simulink library "mobileRoboticsTrainingLib"  (R2017a)
settings: Solver=FixedStepDiscrete  StartTime=0.0  StopTime=10.0  FixedStep=0.01  RelTol=1e-3
values from neighbouring files (symbols this model uses):
  lineLength = xAxesLim(2)/15    [setupRobotSim.m]
  mapForSim = evalin('base',mapVar)    [setStartingPoint.m]    (also in setupRobotSim.m)
undefined symbols (not defined in the file or in its folder): DiscIntNeverNeededParam
libraries: cstblocks x1, simulink_extras x1, simulink x1
settings Model: Creator=sseshadr  LastModifiedBy=sseshadr

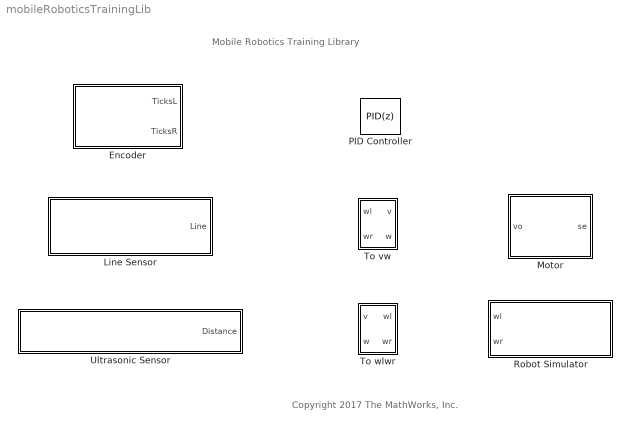
== system mobileRoboticsTrainingLib ==
  note: Mobile Robotics Training Library
  note: Copyright 2017 The MathWorks, Inc.
  Encoder : Subsystem  mask(Encoder Simulation){axleLength=0.1, wheelR=0.05, ticksPerRot=1}
      mask prompts: axleLength "Axle Length (m)"; wheelR "Wheel Radius (m)"; ticksPerRot "Ticks per Rotation"
      mask help:
      | Measure the rotation of left and right motors in ticks.
      |
      | 1 rotation = Number of ticks as specified by the Ticks per Rotation parameter described below.
      |
      | The block outputs a tick count for both a left and a right motor. The tick count:
      | Increments for Clockwise rotation
      | Decrements for Counter-Clockwise rotation
      mask Help: web('Encoder Simulation.htm')
      mask Display: disp('Encoder Simulation')
  Line Sensor : Subsystem  mask(Line Sensor Simulation){mapVariable=mapForSim, envVal=2850, lineVal=2950, sensOff=[0.01 0]}
      mask prompts: mapVariable "Map Variable"; envVal "Environment Value"; lineVal "Line Value"; sensOff "Sensor Offset (m)"
      mask help: Use a simulation map to compute line sensor values based on robot position and sensor offsets.
      mask Help: web('Line Sensor Simulation.htm')
      mask Display: disp('Line Sensor Simulation')
  Motor : Subsystem  mask(Motor Model){motorPlant=1, sensorType=Speed}
      mask prompts: motorPlant "Motor Model"; sensorType "Sensor Type"
      mask help: Use LTI systems to model motors obtained through workflows such as the System Identification App.
      mask Help: web('Motor.htm')
      mask TypeOptions sensorType: Speed | Position
      mask Display:
      | img = imread('motorMask.png');
      | image(img)
  PID Controller : simulink/Continuous/PID Controller  Controller=PID  TimeDomain=Discrete-time  SampleTime=-1  IntegratorMethod=Forward Euler  FilterMethod=Forward Euler  Form=Parallel  UseFilter=on  ControllerParametersSource=internal  P=1  I=1  D=0  N=100  InitialConditionSource=internal  InitialConditionForIntegrator=0  InitialConditionForFilter=0  ExternalReset=none  LimitOutput=off  UpperSaturationLimit=inf  LowerSaturationLimit=-inf  LinearizeAsGain=on  AntiWindupMode=none  Kb=1  TrackingMode=off  Kt=1  PParamMin=[]  PParamMax=[]  IParamMin=[]  IParamMax=[]  DParamMin=[]  DParamMax=[]  NParamMin=[]  NParamMax=[]  KbParamMin=[]  KbParamMax=[]  KtParamMin=[]  KtParamMax=[]  POutMin=[]  POutMax=[]  IOutMin=[]  IOutMax=[]  DOutMin=[]  DOutMax=[]  NOutMin=[]  NOutMax=[]  KbOutMin=[]  KbOutMax=[]  KtOutMin=[]  KtOutMax=[]  IntegratorOutMin=[]  IntegratorOutMax=[]  FilterOutMin=[]  FilterOutMax=[]  SumOutMin=[]  SumOutMax=[]  SumI1OutMin=[]  SumI1OutMax=[]  SumI2OutMin=[]  SumI2OutMax=[]  SumI3OutMin=[]  SumI3OutMax=[]  SumDOutMin=[]  SumDOutMax=[]  SaturationOutMin=[]  SaturationOutMax=[]  IntegratorContinuousStateAttributes=''  IntegratorStateMustResolveToSignalObject=off  IntegratorRTWStateStorageClass=Auto  FilterContinuousStateAttributes=''  FilterStateMustResolveToSignalObject=off  FilterRTWStateStorageClass=Auto  DifferentiatorICPrevScaledInput=0  DifferentiatorOutMin=[]  DifferentiatorOutMax=[]  InitialConditionSetting=Output
  Robot Simulator : Subsystem  Priority=99  mask(Robot Simulator){mapVar=[], startX=1, startY=1, startTheta=0, axleLength=0.1, wheelR=0.05}
      mask prompts: mapVar "Map Variable"; startX "Start X (m)"; startY "Start Y (m)"; startTheta "Theta (deg)"; axleLength "Axle Length (m)"; wheelR "Wheel Radius (m)"
      mask help: Configure robot simulator to use custom simulation maps and simulate closed-loop mobile robotics systems along with appropriate sensor simulation blocks.
      mask init:
      | set_param(bdroot,'SolverType','Fixed-Step');
      | set_param(bdroot,'Solver','FixedStepDiscrete');
      | 
      | if (exist('Ts'))
      |     set_param(bdroot,'FixedStep','Ts');
      | else
      |     set_param(bdroot,'FixedStep','0.01');
      | end
      | 
      | h = findobj('Name','Robot Simulator');
      | if ~isempty(h)
      |     close (h);
      | end
      | setupRobotSim();
      mask Help: web('Robot Simulator.htm')
      mask DialogControl setPos Prompt: Set position interactively
      mask DialogControl setPos Callback:
      | %% Set starting point
      | setStartingPoint();
      mask Display: disp('Robot Simulator')
  To vw : Subsystem  mask(To vw){axleLength=0.1, wheelR=0.05}
      mask prompts: axleLength "Axle Length (m)"; wheelR "Wheel Radius (m)"
      mask help: Converts left (wl) and right (wr) wheel angular velocities into robot linear (v) and angular (w) velocities using robot parameters.
      mask Help: web('To vw.htm')
  To wlwr : Subsystem  mask(To wlwr){axleLength=0.1, wheelR=0.05}
      mask prompts: axleLength "Axle Length (m)"; wheelR "Wheel Radius (m)"
      mask help: Converts robot linear (v) and angular (w) velocities into left (wl) and right (wr) wheel angular velocities using robot parameters.
      mask Help: web('To wlwr.htm')
  Ultrasonic Sensor : Subsystem  mask(Ultrasonic Sensor Simulation){mapVar=mapForSim, maxSenRange=2, minSenRange=0.02, senRes=0.01, sensOff=[0 0]}
      mask prompts: mapVar "Map Variable"; maxSenRange "Maximum Range (m)"; minSenRange "Minimum Range (m)"; senRes "Resolution (m)"; sensOff "Sensor Offset (m)"
      mask help: Use a simulation map to compute ultrasonic sensor values based on robot position and sensor offsets.
      mask init:
      | % %% Read image
      | % imgName = get_param(gcb,'mapFilename');
      | % imgName(1) = []; %Remove extra quotes
      | % imgName(end) = []; %Remove extra quotes
      | % img = imread(imgName);
      | % [imgSize(1),imgSize(2),~] = size(img);
      | % trackSize = str2num(get_param(gcb,'trackSize'));
      | % scaleFactor = imgSize(1)/trackSize(1);
      mask Help: web('Ultrasonic Sensor Simulation.htm')
      mask Display: disp('Ultrasonic Sensor Simulation')

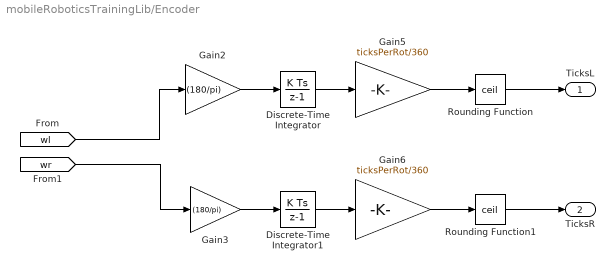
== system mobileRoboticsTrainingLib/Encoder ==
  Discrete-Time Integrator : DiscreteIntegrator  InitialConditionSetting=State (most efficient)  SampleTime=-1  ICPrevOutput=DiscIntNeverNeededParam  ICPrevScaledInput=DiscIntNeverNeededParam
  Discrete-Time Integrator1 : DiscreteIntegrator  InitialConditionSetting=State (most efficient)  SampleTime=-1  ICPrevOutput=DiscIntNeverNeededParam  ICPrevScaledInput=DiscIntNeverNeededParam
  Gain2 : Gain  Gain=(180/pi)
  Gain3 : Gain  Gain=(180/pi)
  Gain5 : Gain  Gain=ticksPerRot/360
  Gain6 : Gain  Gain=ticksPerRot/360
  Rounding Function : Rounding  Operator=ceil
  Rounding Function1 : Rounding  Operator=ceil
  TicksL : Outport
  TicksR : Outport  Port=2
  wires:
  Gain2/1 -> Discrete-Time Integrator/1
  Discrete-Time Integrator1/1 -> Gain6/1
  Gain3/1 -> Discrete-Time Integrator1/1
  Discrete-Time Integrator/1 -> Gain5/1
  Gain5/1 -> Rounding Function/1
  [wr] -> Gain3/1
  [wl] -> Gain2/1
  Gain6/1 -> Rounding Function1/1
  Rounding Function1/1 -> TicksR/1
  Rounding Function/1 -> TicksL/1

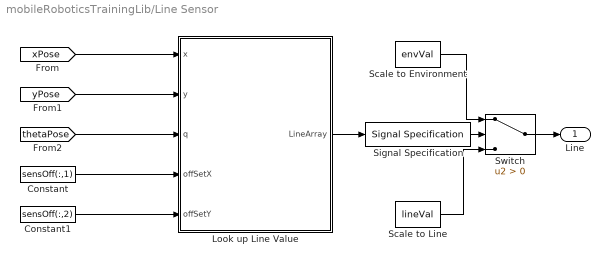
== system mobileRoboticsTrainingLib/Line Sensor ==
  Constant : Constant  Value=sensOff(:,1)
  Constant1 : Constant  Value=sensOff(:,2)
  Look up Line Value : Subsystem
  Scale to Environment : Constant  Value=envVal
  Scale to Line : Constant  Value=lineVal
  Signal Specification : SignalSpecification  Dimensions=length(sensOff(:,1))
  Switch : Switch  Criteria=u2 > Threshold
  Line : Outport
  wires:
  [thetaPose] -> Look up Line Value/3(q)
  [yPose] -> Look up Line Value/2(y)
  [xPose] -> Look up Line Value/1(x)
  Scale to Line/1 -> Switch/3
  Scale to Environment/1 -> Switch/1
  Switch/1 -> Line/1
  Constant/1 -> Look up Line Value/4(offSetX)
  Constant1/1 -> Look up Line Value/5(offSetY)
  Look up Line Value/1(LineArray) -> Signal Specification/1
  Signal Specification/1 -> Switch/2

== system mobileRoboticsTrainingLib/Motor ==
  vo : Inport
  Constant : Constant  Value=sensorType
  Discrete-Time Integrator : DiscreteIntegrator  InitialConditionSetting=State (most efficient)  SampleTime=-1  ICPrevOutput=DiscIntNeverNeededParam  ICPrevScaledInput=DiscIntNeverNeededParam
  Motor : cstblocks/LTI System  sys=motorPlant  IC=[]
  Radians to Degrees : simulink_extras/Transformations/Radians to Degrees
  Switch : Switch  Criteria=u2 > Threshold  Threshold=1
  se : Outport
  wires:
  Radians to Degrees/1 -> Switch/1
  Discrete-Time Integrator/1 -> Radians to Degrees/1
  Constant/1 -> Switch/2
  vo/1 -> Motor/1
  Switch/1 -> se/1
  Motor/1 -> Discrete-Time Integrator/1, Switch/3

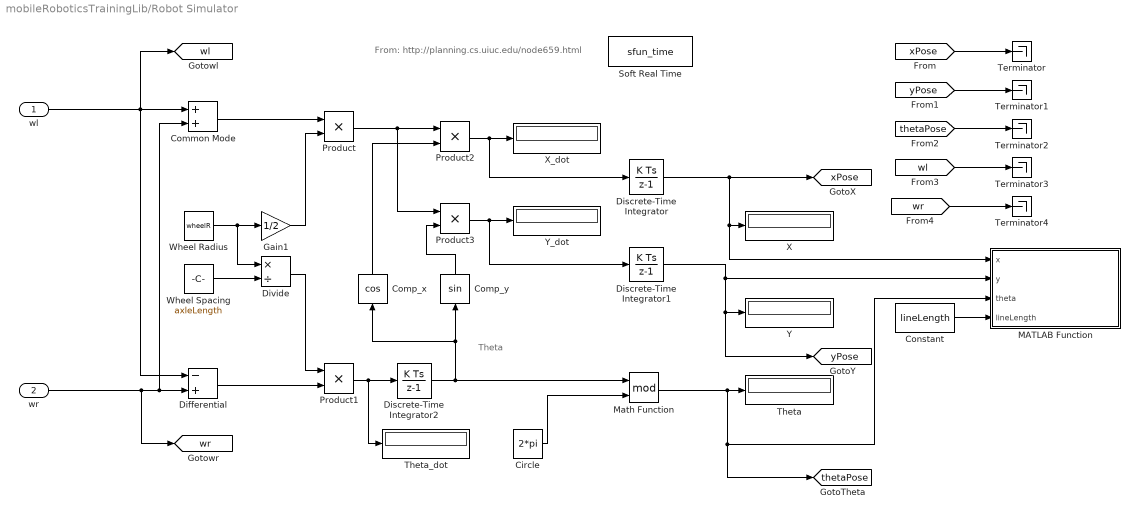
== system mobileRoboticsTrainingLib/Robot Simulator ==
  note: From: http://planning.cs.uiuc.edu/node659.html
  note: Theta
  wl : Inport
  wr : Inport  Port=2
  Circle : Constant  Value=2*pi
  Common Mode : Sum
  Comp_x : Trigonometry  Operator=cos
  Comp_y : Trigonometry
  Constant : Constant  Value=lineLength
  Differential : Sum  Inputs=-+
  Discrete-Time Integrator : DiscreteIntegrator  InitialCondition=startX  InitialConditionSetting=State (most efficient)  SampleTime=-1  ICPrevOutput=DiscIntNeverNeededParam  ICPrevScaledInput=DiscIntNeverNeededParam
  Discrete-Time Integrator1 : DiscreteIntegrator  InitialCondition=startY  InitialConditionSetting=State (most efficient)  SampleTime=-1  ICPrevOutput=DiscIntNeverNeededParam  ICPrevScaledInput=DiscIntNeverNeededParam
  Discrete-Time Integrator2 : DiscreteIntegrator  InitialCondition=startTheta*(pi/180)  InitialConditionSetting=State (most efficient)  SampleTime=-1  ICPrevOutput=DiscIntNeverNeededParam  ICPrevScaledInput=DiscIntNeverNeededParam
  Divide : Product  Inputs=*/
  Gain1 : Gain  Gain=1/2
  MATLAB Function : MATLAB Function  TreatAsAtomicUnit=on
  Math Function : Math  Operator=mod  SaturateOnIntegerOverflow=on
  Product{,1..3} (4 alike) : Product  RndMeth=Zero
  Soft Real Time : S-Function  FunctionName=sfun_time  Parameters=x  SFunctionDeploymentMode=off  EnableBusSupport=off  mask{x=1}
      mask prompts: x "Time Scaling Factor"
      mask Display:
      | color('red')
      | disp('Soft Real Time')
  Terminator{,1..4} (5 alike) : Terminator
  Theta : Display
  Theta_dot : Display
  Wheel Radius : Constant  Value=wheelR
  Wheel Spacing : Constant  Value=axleLength
  X : Display
  X_dot : Display
  Y : Display
  Y_dot : Display
  tag scope: thetaPose=global, wl=global, wr=global, xPose=global, yPose=global
  wires:
  [thetaPose] -> Terminator2/1
  [yPose] -> Terminator1/1
  [xPose] -> Terminator/1
  Constant/1 -> MATLAB Function/4(lineLength)
  Circle/1 -> Math Function/2
  Product/1 -> Product2/1, Product3/1
  Common Mode/1 -> Product/1
  Gain1/1 -> Product/2
  Product2/1 -> X_dot/1, Discrete-Time Integrator/1
  Wheel Spacing/1 -> Divide/2
  Wheel Radius/1 -> Gain1/1, Divide/1
  Product1/1 -> Theta_dot/1, Discrete-Time Integrator2/1
  Comp_x/1 -> Product2/2
  wl/1 -> Differential/1, Common Mode/1, [wl]
  Discrete-Time Integrator2/1 -> Comp_y/1, Comp_x/1, Math Function/1
  wr/1 -> Differential/2, Common Mode/2, [wr]
  Divide/1 -> Product1/1
  Discrete-Time Integrator1/1 -> MATLAB Function/2(y), [yPose], Y/1
  Product3/1 -> Y_dot/1, Discrete-Time Integrator1/1
  Discrete-Time Integrator/1 -> X/1, MATLAB Function/1(x), [xPose]
  Comp_y/1 -> Product3/2
  Differential/1 -> Product1/2
  Math Function/1 -> Theta/1, MATLAB Function/3(theta), [thetaPose]
  [wl] -> Terminator3/1
  [wr] -> Terminator4/1

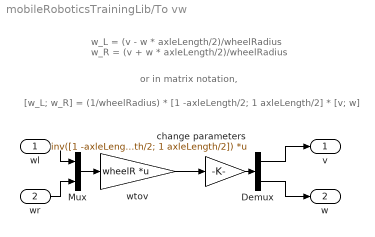
== system mobileRoboticsTrainingLib/To vw ==
  note: [w_L; w_R] = (1/wheelRadius) * [1 -axleLength/2; 1 axleLength/2] * [v; w]
  note: w_L  = (v - w * axleLength/2)/wheelRadius
      | w_R = (v + w * axleLength/2)/wheelRadius
  note: or in matrix notation,
  wl : Inport
  wr : Inport  Port=2
  Demux : Demux  Outputs=2
  Mux : Mux  Inputs=2
  change parameters : Gain  Gain=inv([1 -axleLength/2; 1 axleLength/2])  Multiplication=Matrix(K*u)
  wtov : Gain  Gain=wheelR  Multiplication=Matrix(K*u)
  v : Outport
  w : Outport  Port=2
  wires:
  Demux/2 -> w/1
  Demux/1 -> v/1
  wl/1 -> Mux/1
  wr/1 -> Mux/2
  Mux/1 -> wtov/1
  change parameters/1 -> Demux/1
  wtov/1 -> change parameters/1

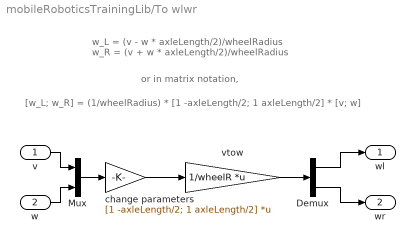
== system mobileRoboticsTrainingLib/To wlwr ==
  note: [w_L; w_R] = (1/wheelRadius) * [1 -axleLength/2; 1 axleLength/2] * [v; w]
  note: w_L  = (v - w * axleLength/2)/wheelRadius
      | w_R = (v + w * axleLength/2)/wheelRadius
  note: or in matrix notation,
  v : Inport
  w : Inport  Port=2
  Demux : Demux  Outputs=2
  Mux : Mux  Inputs=2
  change parameters : Gain  Gain=[1 -axleLength/2; 1 axleLength/2]  Multiplication=Matrix(K*u)
  vtow : Gain  Gain=1/wheelR  Multiplication=Matrix(K*u)
  wl : Outport
  wr : Outport  Port=2
  wires:
  Mux/1 -> change parameters/1
  w/1 -> Mux/2
  v/1 -> Mux/1
  Demux/1 -> wl/1
  Demux/2 -> wr/1
  change parameters/1 -> vtow/1
  vtow/1 -> Demux/1

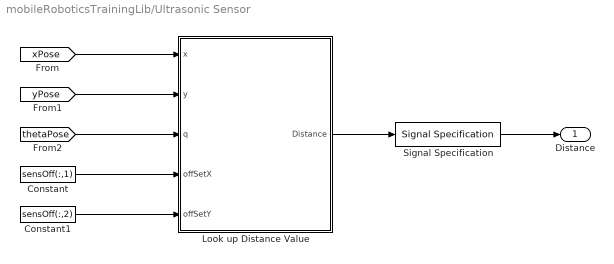
== system mobileRoboticsTrainingLib/Ultrasonic Sensor ==
  Constant : Constant  Value=sensOff(:,1)
  Constant1 : Constant  Value=sensOff(:,2)
  Look up Distance Value : Subsystem
  Signal Specification : SignalSpecification  Dimensions=length(sensOff(:,1))
  Distance : Outport
  wires:
  [thetaPose] -> Look up Distance Value/3(q)
  [xPose] -> Look up Distance Value/1(x)
  [yPose] -> Look up Distance Value/2(y)
  Constant1/1 -> Look up Distance Value/5(offSetY)
  Constant/1 -> Look up Distance Value/4(offSetX)
  Look up Distance Value/1(Distance) -> Signal Specification/1
  Signal Specification/1 -> Distance/1

== system mobileRoboticsTrainingLib/Line Sensor/Look up Line Value ==
  x : Inport
  y : Inport  Port=2
  q : Inport  Port=3
  offSetX : Inport  Port=4
  offSetY : Inport  Port=5
  For Each Subsystem : Subsystem  TreatAsAtomicUnit=on
  LineArray : Outport
  wires:
  x/1 -> For Each Subsystem/1(x)
  y/1 -> For Each Subsystem/2(y)
  offSetX/1 -> For Each Subsystem/4(offSetX)
  q/1 -> For Each Subsystem/3(q)
  offSetY/1 -> For Each Subsystem/5(offSetY)
  For Each Subsystem/1(LineArray) -> LineArray/1

== system mobileRoboticsTrainingLib/Ultrasonic Sensor/Look up Distance Value ==
  x : Inport
  y : Inport  Port=2
  q : Inport  Port=3
  offSetX : Inport  Port=4
  offSetY : Inport  Port=5
  Calculate Rotation Matrix : MATLAB Function  TreatAsAtomicUnit=on
  Subsystem : Subsystem
  Distance : Outport
  wires:
  q/1 -> Calculate Rotation Matrix/1(q)
  Subsystem/1(DistanceArray) -> Distance/1
  Calculate Rotation Matrix/1(rotMat) -> Subsystem/3(R)
  y/1 -> Subsystem/5(y)
  x/1 -> Subsystem/4(x)
  offSetY/1 -> Subsystem/2(offSetY)
  offSetX/1 -> Subsystem/1(offSetX)

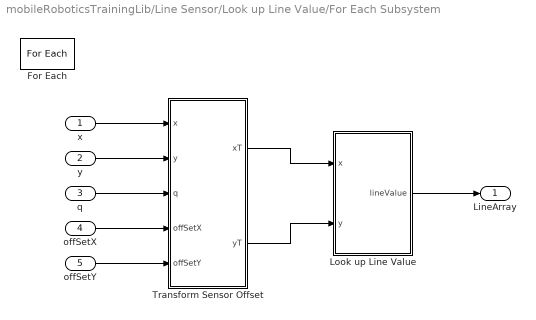
== system mobileRoboticsTrainingLib/Line Sensor/Look up Line Value/For Each Subsystem ==
  x : Inport
  y : Inport  Port=2
  q : Inport  Port=3
  offSetX : Inport  Port=4  Partition=on  PartitionDimension=1  PartitionWidth=1
  offSetY : Inport  Port=5  Partition=on  PartitionDimension=1  PartitionWidth=1
  For Each : ForEach  DisableCoverage=on  IndexMode=One-based
  Look up Line Value : Subsystem  TreatAsAtomicUnit=on
  Transform Sensor Offset : MATLAB Function  TreatAsAtomicUnit=on
  LineArray : Outport  ConcatenationDimension=1
  wires:
  Look up Line Value/1(lineValue) -> LineArray/1
  Transform Sensor Offset/1(xT) -> Look up Line Value/1(x)
  Transform Sensor Offset/2(yT) -> Look up Line Value/2(y)
  offSetX/1 -> Transform Sensor Offset/4(offSetX)
  offSetY/1 -> Transform Sensor Offset/5(offSetY)
  x/1 -> Transform Sensor Offset/1(x)
  y/1 -> Transform Sensor Offset/2(y)
  q/1 -> Transform Sensor Offset/3(q)

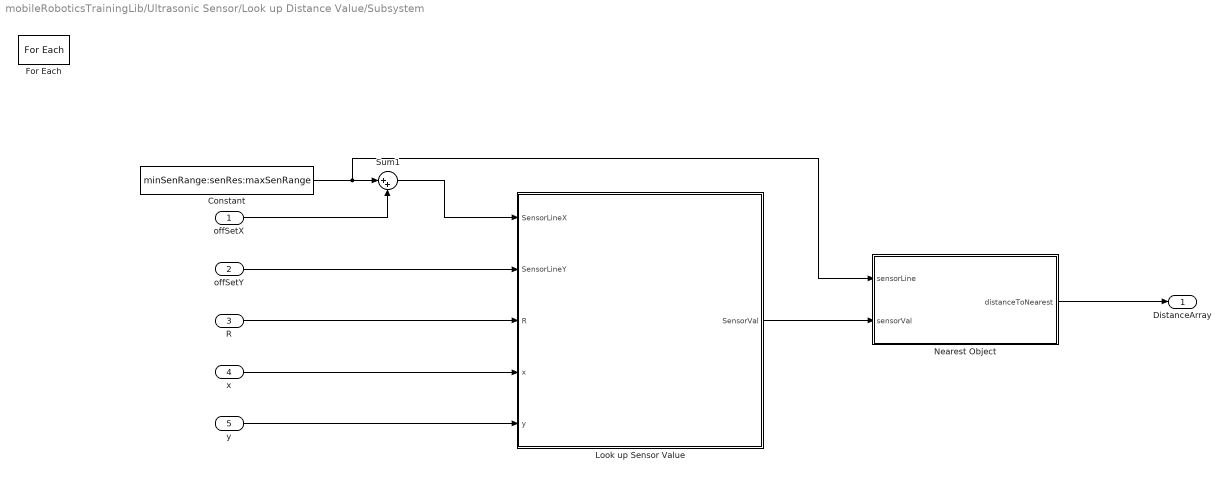
== system mobileRoboticsTrainingLib/Ultrasonic Sensor/Look up Distance Value/Subsystem ==
  offSetX : Inport  Partition=on  PartitionDimension=1  PartitionWidth=1
  offSetY : Inport  Port=2  Partition=on  PartitionDimension=1  PartitionWidth=1
  R : Inport  Port=3
  x : Inport  Port=4
  y : Inport  Port=5
  Constant : Constant  Value=minSenRange:senRes:maxSenRange
  For Each : ForEach  DisableCoverage=on  IndexMode=One-based
  Look up Sensor Value : Subsystem  TreatAsAtomicUnit=on
  Nearest Object : MATLAB Function  TreatAsAtomicUnit=on
  Sum1 : Sum  Inputs=|++
  DistanceArray : Outport  ConcatenationDimension=1
  wires:
  Nearest Object/1(distanceToNearest) -> DistanceArray/1
  Look up Sensor Value/1(SensorVal) -> Nearest Object/2(sensorVal)
  y/1 -> Look up Sensor Value/5(y)
  x/1 -> Look up Sensor Value/4(x)
  R/1 -> Look up Sensor Value/3(R)
  offSetY/1 -> Look up Sensor Value/2(SensorLineY)
  Sum1/1 -> Look up Sensor Value/1(SensorLineX)
  offSetX/1 -> Sum1/2
  Constant/1 -> Nearest Object/1(sensorLine), Sum1/1

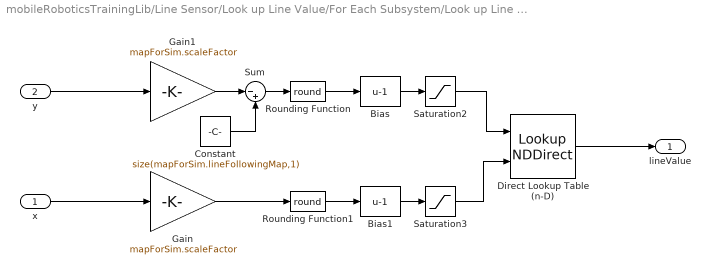
== system mobileRoboticsTrainingLib/Line Sensor/Look up Line Value/For Each Subsystem/Look up Line Value ==
  x : Inport
  y : Inport  Port=2
  Bias : Bias  Bias=-1
  Bias1 : Bias  Bias=-1
  Constant : Constant  Value=size(mapForSim.lineFollowingMap,1)
  Direct Lookup Table (n-D) : LookupNDDirect  Table=mapForSim.lineFollowingMap  DiagnosticForOutOfRangeInput=Error
  Gain : Gain  Gain=mapForSim.scaleFactor
  Gain1 : Gain  Gain=mapForSim.scaleFactor
  Rounding Function : Rounding  Operator=round
  Rounding Function1 : Rounding  Operator=round
  Saturation2 : Saturate  UpperLimit=size(mapForSim.lineFollowingMap,1)-1  LowerLimit=0
  Saturation3 : Saturate  UpperLimit=size(mapForSim.lineFollowingMap,2)-1  LowerLimit=0
  Sum : Sum  Inputs=|-+
  lineValue : Outport
  wires:
  Saturation3/1 -> Direct Lookup Table (n-D)/2
  Saturation2/1 -> Direct Lookup Table (n-D)/1
  Rounding Function1/1 -> Bias1/1
  Rounding Function/1 -> Bias/1
  Bias/1 -> Saturation2/1
  Bias1/1 -> Saturation3/1
  Direct Lookup Table (n-D)/1 -> lineValue/1
  Constant/1 -> Sum/2
  Gain1/1 -> Sum/1
  Sum/1 -> Rounding Function/1
  x/1 -> Gain/1
  y/1 -> Gain1/1
  Gain/1 -> Rounding Function1/1

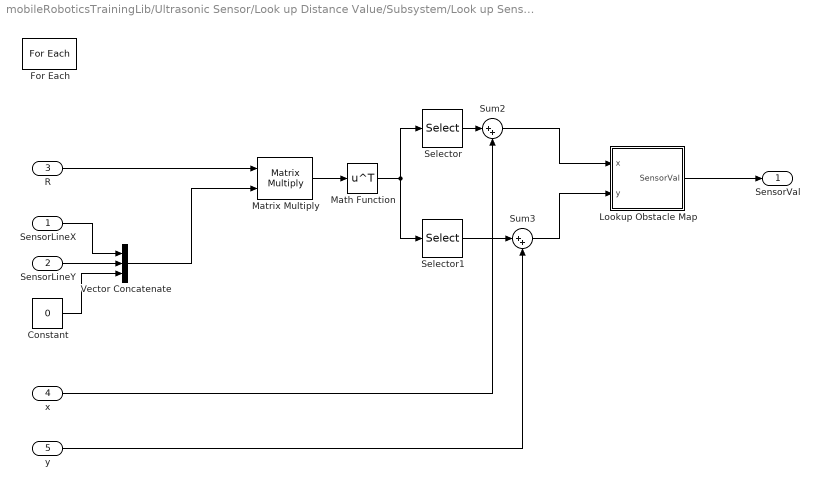
== system mobileRoboticsTrainingLib/Ultrasonic Sensor/Look up Distance Value/Subsystem/Look up Sensor Value ==
  SensorLineX : Inport  Partition=on  PartitionDimension=1  PartitionWidth=1
  SensorLineY : Inport  Port=2
  R : Inport  Port=3
  x : Inport  Port=4
  y : Inport  Port=5
  Constant : Constant  Value=0
  For Each : ForEach  DisableCoverage=on  IndexMode=One-based
  Lookup Obstacle Map : Subsystem
  Math Function : Math  Operator=transpose  SaturateOnIntegerOverflow=on
  Matrix Multiply : Product  Multiplication=Matrix(*)
  Selector : Selector  InputPortWidth=3  IndexOptions=Index vector (dialog)  Indices=1  OutputSizes=1
  Selector1 : Selector  InputPortWidth=3  IndexOptions=Index vector (dialog)  Indices=[2]  OutputSizes=1
  Sum2 : Sum  Inputs=|++
  Sum3 : Sum  Inputs=|++
  Vector Concatenate : Concatenate  NumInputs=3  Mode=Multidimensional array
  SensorVal : Outport  ConcatenationDimension=1
  wires:
  SensorLineX/1 -> Vector Concatenate/1
  SensorLineY/1 -> Vector Concatenate/2
  Constant/1 -> Vector Concatenate/3
  R/1 -> Matrix Multiply/1
  Vector Concatenate/1 -> Matrix Multiply/2
  Matrix Multiply/1 -> Math Function/1
  Math Function/1 -> Selector1/1, Selector/1
  Selector/1 -> Sum2/1
  Sum2/1 -> Lookup Obstacle Map/1(x)
  x/1 -> Sum2/2
  Selector1/1 -> Sum3/1
  y/1 -> Sum3/2
  Lookup Obstacle Map/1(SensorVal) -> SensorVal/1
  Sum3/1 -> Lookup Obstacle Map/2(y)

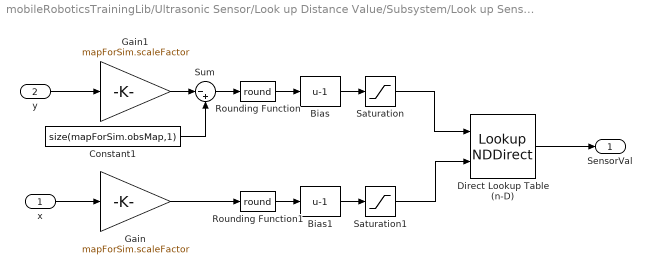
== system mobileRoboticsTrainingLib/Ultrasonic Sensor/Look up Distance Value/Subsystem/Look up Sensor Value/Lookup Obstacle Map ==
  x : Inport
  y : Inport  Port=2
  Bias : Bias  Bias=-1
  Bias1 : Bias  Bias=-1
  Constant1 : Constant  Value=size(mapForSim.obsMap,1)
  Direct Lookup Table (n-D) : LookupNDDirect  Table=mapForSim.obsMap  DiagnosticForOutOfRangeInput=Error
  Gain : Gain  Gain=mapForSim.scaleFactor
  Gain1 : Gain  Gain=mapForSim.scaleFactor
  Rounding Function : Rounding  Operator=round
  Rounding Function1 : Rounding  Operator=round
  Saturation : Saturate  UpperLimit=size(mapForSim.obsMap,1)-1  LowerLimit=0
  Saturation1 : Saturate  UpperLimit=size(mapForSim.obsMap,2)-1  LowerLimit=0
  Sum : Sum  Inputs=|-+
  SensorVal : Outport
  wires:
  Bias1/1 -> Saturation1/1
  Bias/1 -> Saturation/1
  y/1 -> Gain1/1
  Rounding Function/1 -> Bias/1
  Gain/1 -> Rounding Function1/1
  x/1 -> Gain/1
  Rounding Function1/1 -> Bias1/1
  Sum/1 -> Rounding Function/1
  Gain1/1 -> Sum/1
  Constant1/1 -> Sum/2
  Direct Lookup Table (n-D)/1 -> SensorVal/1
  Saturation/1 -> Direct Lookup Table (n-D)/1
  Saturation1/1 -> Direct Lookup Table (n-D)/2

== matlab function mobileRoboticsTrainingLib/Robot Simulator/MATLAB Function ==
  data: x input; y input; theta input; lineLength input
function plotRobot(x,y,theta,lineLength)
% Get plot details
coder.extrinsic('evalin','plot')
ph1 = evalin('base','PlotHandle1');
ph2 = evalin('base','PlotHandle2');

% Find length orientation line
xp = [x x+lineLength*cos(theta)];
yp = [y y+lineLength*sin(theta)];

% Plot robot
set(ph1,'xdata',xp,'ydata',yp);
set(ph2,'xdata',x,'ydata',y);
drawnow('limitrate')

== matlab function mobileRoboticsTrainingLib/Line Sensor/Look up Line Value/For Each Subsystem/Transform Sensor Offset ==
  data: x input; xT output; y input; q input; yT output; offSetX input; offSetY input
function [xT,yT] = transformPoints(x,y,q,offSetX,offSetY)

theta = q;

rotMat = [cos(theta) -sin(theta) 0;
          sin(theta)  cos(theta) 0;
          0           0          1];

transPt = rotMat * [offSetX;offSetY;0];

xT = x + transPt(1);
yT = y + transPt(2);
    
end

== matlab function mobileRoboticsTrainingLib/Ultrasonic Sensor/Look up Distance Value/Calculate Rotation Matrix ==
  data: rotMat output; q input
function rotMat = calcRotMat(q)

theta = q;

rotMat = [cos(theta) -sin(theta) 0;
          sin(theta)  cos(theta) 0;
          0           0          1];
    
end

== matlab function mobileRoboticsTrainingLib/Ultrasonic Sensor/Look up Distance Value/Subsystem/Nearest Object ==
  data: sensorLine input; sensorVal input; distanceToNearest output
function distanceToNearest = nearestObject(sensorLine,sensorVal)

%Find the first 'hit' in Sensor Line
nearestIdx = find(~sensorVal,1,'first');

distanceToNearest = 0;

if (~isempty(nearestIdx))
    distanceToNearest = sensorLine(nearestIdx(1));
end

end
